simulink model "stepinputresponse"  (R2022b)
settings: Solver=VariableStepAuto  StartTime=0.0  StopTime=120  RelTol=1e-3
libraries: simulink x1
settings Model: Creator=Asus  LastModifiedBy=Asus

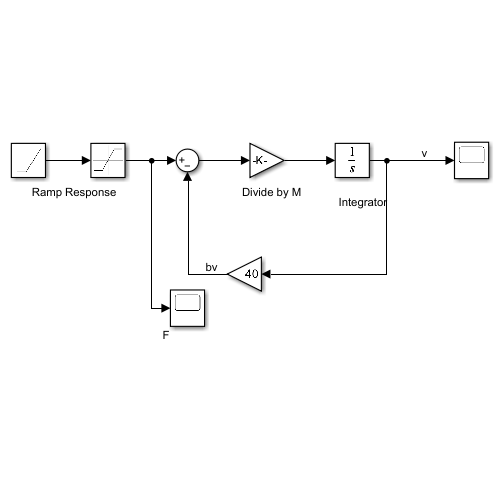
[thumbnail: Simulink's stored preview of the top-level diagram]
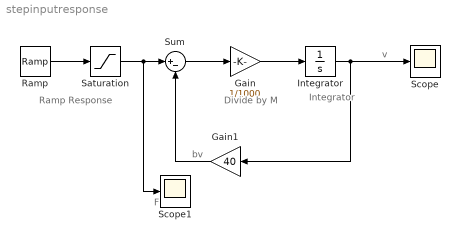
== system stepinputresponse ==
  note: Ramp Response
  note: Divide by M
  note: v
  note: bv
  note: F
  note: Integrator
  Gain : Gain  Gain=1/1000
  Gain1 : Gain  Gain=40
  Integrator : Integrator
  Ramp : simulink/Sources/Ramp  slope=80  start=0  InitialOutput=0
  Saturation : Saturate  UpperLimit=2000
  Scope : Scope
  Scope1 : Scope
  Sum : Sum  Inputs=|+-
  wires:
  Gain/1 -> Integrator/1
  Integrator/1 -> Gain1/1, Scope/1
  Gain1/1 -> Sum/2
  Sum/1 -> Gain/1
  Ramp/1 -> Saturation/1
  Saturation/1 -> Scope1/1, Sum/1
